simulink model "cacadeculo"  (R2014a)
settings: Solver=ode45  StartTime=0.0  StopTime=10.0  RelTol=1e-3
undefined symbols (not defined in the file): B, K, Kd, m
settings Model: Creator=Manuel  LastModifiedBy=Manuel

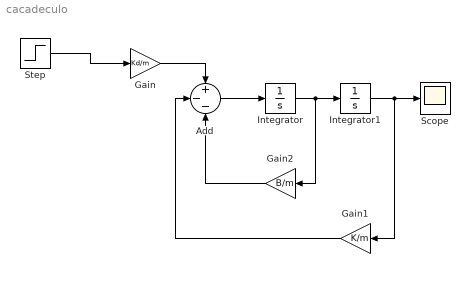
== system cacadeculo ==
  Add : Sum  Inputs=+--
  Gain : Gain  Gain=Kd/m
  Gain1 : Gain  Gain=K/m
  Gain2 : Gain  Gain=B/m
  Integrator : Integrator
  Integrator1 : Integrator
  Scope : Scope
  Step : Step  After=0.1  SampleTime=0
  wires:
  Step/1 -> Gain/1
  Gain/1 -> Add/1
  Add/1 -> Integrator/1
  Integrator/1 -> Gain2/1, Integrator1/1
  Integrator1/1 -> Gain1/1, Scope/1
  Gain1/1 -> Add/2
  Gain2/1 -> Add/3
